simulink model "lab1_sum_constant_display"  (R2019a)
settings: Solver=VariableStepAuto  StartTime=0.0  StopTime=10.0  RelTol=1e-3
settings Model: Creator=LEGION  LastModifiedBy=LEGION

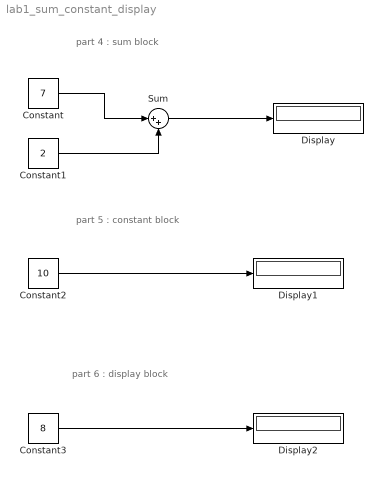
== system lab1_sum_constant_display ==
  note: part 4 : sum block
  note: part 5 : constant block
  note: part 6 : display block
  Constant : Constant  Value=7
  Constant1 : Constant  Value=2
  Constant2 : Constant  Value=10
  Constant3 : Constant  Value=8
  Display : Display
  Display1 : Display
  Display2 : Display
  Sum : Sum  Inputs=|++
  wires:
  Sum/1 -> Display/1
  Constant/1 -> Sum/1
  Constant1/1 -> Sum/2
  Constant2/1 -> Display1/1
  Constant3/1 -> Display2/1
